simulink library "devel_lib"  (R2025a)
settings: Solver=VariableStepAuto  StartTime=0.0  StopTime=10.0  RelTol=1e-3
values from neighbouring files (symbols this model uses):
  simstruct = evalin('base', 'simstruct')    [uct_autograder_app.m]
libraries: mmuct_lib x5, simulink x2, dhaouadi2013_lib x2, $bdroot x1
settings Model: Creator=nicolls  LastModifiedBy=nicolls

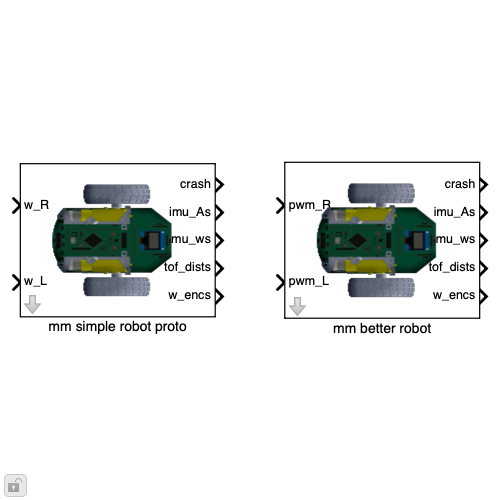
[thumbnail: Simulink's stored preview of the top-level diagram]
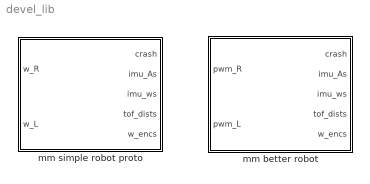
== system devel_lib ==
  mm better robot : Subsystem  mask{simstruct=simstruct, x0=0.1, y0=0.1, theta0=0, motd=0, wav_sd=0, wl_stfrac=0, wr_stfrac=0, as_rot=[0 0 0 0], as_bias=0*[0 0 0], as_sd=0, ws_rot=[0 0 0 0], ws_bias=0*[0 0 0], ws_sd=0, tof_sd=0, enc_sd=0}
      mask prompts: simstruct "Simulation structure variable"; x0 "x0 (m)"; y0 "y0 (m)"; theta0 "theta0 (rad)"; motd "Motor direction (0-3)"; wav_sd "Wheel ang vel stddev"; wl_stfrac "Wheel stutter left (frac)"; wr_stfrac "Wheel stutter right (frac)"; as_rot "as rotation (angle axis)"; as_bias "as bias"; as_sd "as stddev"; ws_rot "ws rotation (angle axis)"; ws_bias "ws bias"; ws_sd "ws stddev"; tof_sd "TOF stddev"; enc_sd "Enc stddev"
      mask DialogControl Container7 Prompt: Initial pose
      mask DialogControl Container3 Prompt: Motor drive variation
      mask DialogControl Container4 Prompt: IMU
      mask DialogControl Container9 Prompt: TOF
      mask DialogControl Container10 Prompt: Wheel encoder
      mask Display: image('uctmm_image.png');
  mm simple robot proto : Subsystem  mask{simstruct=simstruct, x0=0.1, y0=0.1, theta0=0}
      mask prompts: simstruct "Simulation structure variable"; x0 "x0 (m)"; y0 "y0 (m)"; theta0 "theta0 (rad)"
      mask DialogControl Container3 Prompt: Initial pose
      mask Display: image('uctmm_image.png');

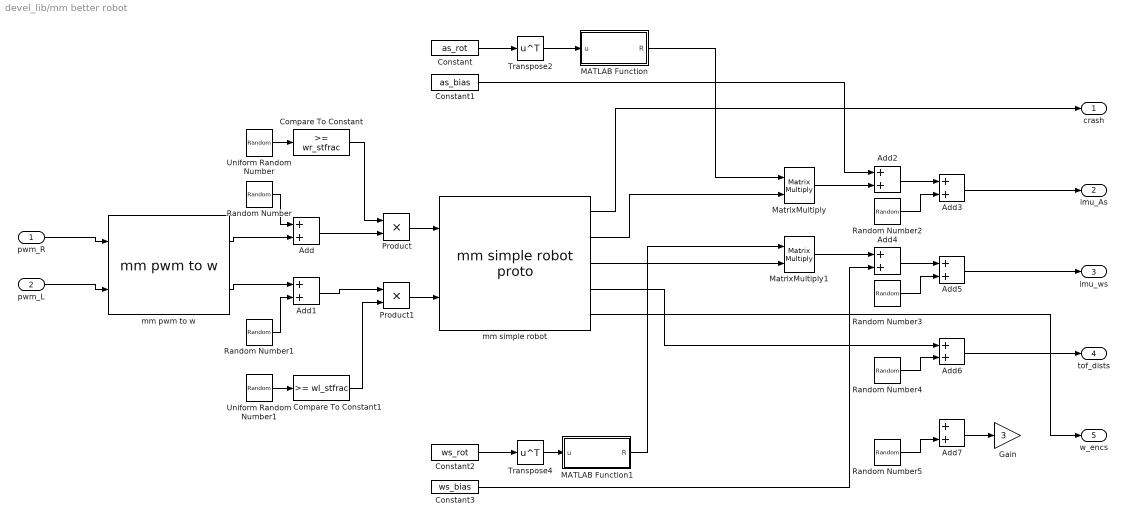
== system devel_lib/mm better robot ==
  pwm_R : Inport
  pwm_L : Inport  Port=2
  Add{,1..7} (8 alike) : Sum
  Compare To Constant : simulink/Logic and Bit Operations/Compare To Constant  relop=>=  const=wr_stfrac  OutDataTypeStr=boolean
  Compare To Constant1 : simulink/Logic and Bit Operations/Compare To Constant  relop=>=  const=wl_stfrac  OutDataTypeStr=boolean
  Constant : Constant  Value=as_rot
  Constant1 : Constant  Value=as_bias
  Constant2 : Constant  Value=ws_rot
  Constant3 : Constant  Value=ws_bias
  Gain : Gain  Gain=3
  MATLAB Function : MATLAB Function  TreatAsAtomicUnit=on
  MATLAB Function1 : MATLAB Function  TreatAsAtomicUnit=on
  MatrixMultiply : Product  Multiplication=Matrix(*)
  MatrixMultiply1 : Product  Multiplication=Matrix(*)
  Product : Product
  Product1 : Product
  Random Number : RandomNumber  Variance=wav_sd^2  SampleTime=0.1
  Random Number1 : RandomNumber  Variance=wav_sd^2  Seed=1  SampleTime=0.1
  Random Number2 : RandomNumber  Variance=as_sd^2  Seed=[10 11 12]  SampleTime=0.1
  Random Number3 : RandomNumber  Variance=ws_sd^2  Seed=[13 14 15]  SampleTime=0.1
  Random Number4 : RandomNumber  Variance=tof_sd^2  Seed=[16 17 18]  SampleTime=0.1
  Random Number5 : RandomNumber  Variance=enc_sd^2  Seed=[19 20]  SampleTime=0.1
  Transpose2 : Math  Operator=transpose
  Transpose4 : Math  Operator=transpose
  Uniform Random Number : UniformRandomNumber  Minimum=0  Seed=3  SampleTime=0.1
  Uniform Random Number1 : UniformRandomNumber  Minimum=0  Seed=2  SampleTime=0.1
  mm pwm to w : mmuct_lib/mm pwm to w  deadb=30  maxw=2*pi  motd=motd
  mm simple robot : $bdroot/mm simple robot proto  simstruct=simstruct  x0=x0  y0=y0  theta0=theta0
  crash : Outport
  imu_As : Outport  Port=2
  imu_ws : Outport  Port=3
  tof_dists : Outport  Port=4
  w_encs : Outport  Port=5
  wires:
  pwm_R/1 -> mm pwm to w/1
  pwm_L/1 -> mm pwm to w/2
  mm pwm to w/1 -> Add/2
  Random Number/1 -> Add/1
  mm pwm to w/2 -> Add1/1
  Random Number1/1 -> Add1/2
  mm simple robot/1 -> crash/1
  Uniform Random Number/1 -> Compare To Constant/1
  Product/1 -> mm simple robot/1
  Add/1 -> Product/2
  Uniform Random Number1/1 -> Compare To Constant1/1
  Product1/1 -> mm simple robot/2
  Compare To Constant1/1 -> Product1/2
  Add1/1 -> Product1/1
  Compare To Constant/1 -> Product/1
  MATLAB Function/1(R) -> MatrixMultiply/1
  MatrixMultiply/1 -> Add2/2
  Add3/1 -> imu_As/1
  Constant2/1 -> Transpose4/1
  MATLAB Function1/1(R) -> MatrixMultiply1/1
  MatrixMultiply1/1 -> Add4/1
  Add4/1 -> Add5/1
  Random Number3/1 -> Add5/2
  Add5/1 -> imu_ws/1
  Random Number4/1 -> Add6/2
  mm simple robot/4 -> Add6/1
  Add6/1 -> tof_dists/1
  Add7/1 -> Gain/1
  Random Number5/1 -> Add7/2
  Constant/1 -> Transpose2/1
  Constant1/1 -> Add2/1
  Constant3/1 -> Add4/2
  mm simple robot/2 -> MatrixMultiply/2
  Transpose4/1 -> MATLAB Function1/1(u)
  mm simple robot/3 -> MatrixMultiply1/2
  Transpose2/1 -> MATLAB Function/1(u)
  Add2/1 -> Add3/1
  Random Number2/1 -> Add3/2
  mm simple robot/5 -> w_encs/1

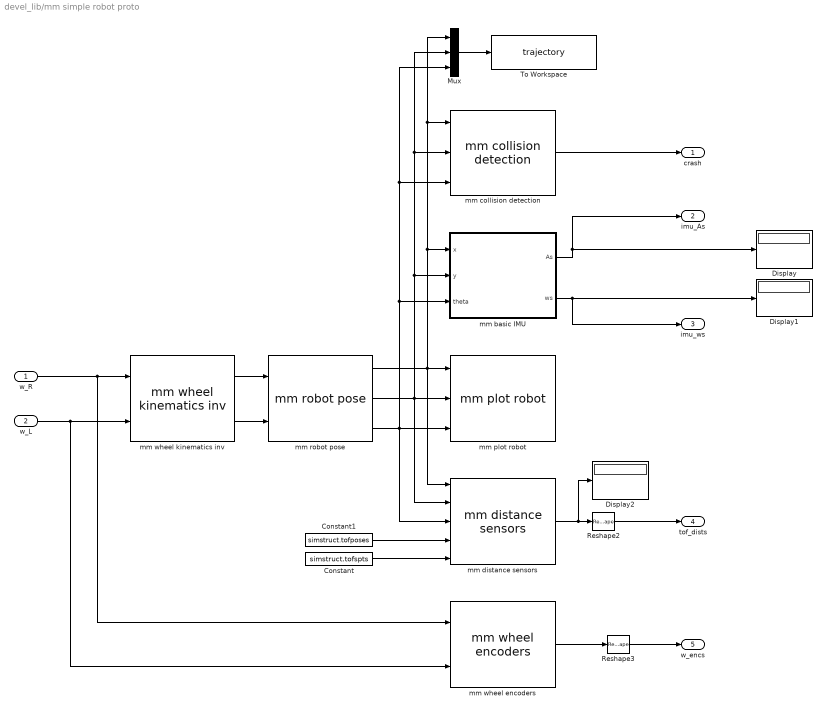
== system devel_lib/mm simple robot proto ==
  w_R : Inport
  w_L : Inport  Port=2
  Constant : Constant  Value=simstruct.tofspts
  Constant1 : Constant  Value=simstruct.tofposes
  Display : Display
  Display1 : Display
  Display2 : Display
  Mux : Mux  Inputs=3
  Reshape2 : Reshape
  Reshape3 : Reshape
  To Workspace : ToWorkspace  VariableName=trajectory  SaveFormat=Timeseries  SampleTime=-1
  mm basic IMU : Subsystem  AncestorBlock=mmuct_lib/mm basic IMU
  mm collision detection : mmuct_lib/mm collision detection  simstruct=simstruct
      settings: SourceProductName=UCT EEE Micromouse
  mm distance sensors : mmuct_lib/mm distance sensors  simstruct=simstruct  debug=0
      settings: SourceProductName=UCT EEE Micromouse
  mm plot robot : mmuct_lib/mm plot robot  simstruct=simstruct  x0=0.1  y0=0.1  theta0=0
      settings: SourceProductName=UCT EEE Micromouse
  mm robot pose : dhaouadi2013_lib/mm robot pose  x0=x0  y0=y0  theta0=0
  mm wheel encoders : mmuct_lib/mm wheel encoders  ticsperrev=8
  mm wheel kinematics inv : dhaouadi2013_lib/mm wheel kinematics inv  L=simstruct.L  R=simstruct.R
  crash : Outport
  imu_As : Outport  Port=2
  imu_ws : Outport  Port=3
  tof_dists : Outport  Port=4
  w_encs : Outport  Port=5
  wires:
  mm basic IMU/2(ws) -> Display1/1, imu_ws/1
  Reshape3/1 -> w_encs/1
  Reshape2/1 -> tof_dists/1
  mm basic IMU/1(As) -> Display/1, imu_As/1
  mm wheel encoders/1 -> Reshape3/1
  mm distance sensors/1 -> Display2/1, Reshape2/1
  Constant/1 -> mm distance sensors/5
  Constant1/1 -> mm distance sensors/4
  mm wheel kinematics inv/2 -> mm robot pose/2
  mm robot pose/2 -> Mux/2, mm collision detection/2, mm basic IMU/2(y), mm distance sensors/2, mm plot robot/2
  mm wheel kinematics inv/1 -> mm robot pose/1
  mm robot pose/1 -> Mux/1, mm collision detection/1, mm basic IMU/1(x), mm plot robot/1, mm distance sensors/1
  mm robot pose/3 -> mm distance sensors/3, Mux/3, mm collision detection/3, mm basic IMU/3(theta), mm plot robot/3
  mm collision detection/1 -> crash/1
  w_L/1 -> mm wheel encoders/2, mm wheel kinematics inv/2
  w_R/1 -> mm wheel encoders/1, mm wheel kinematics inv/1
  Mux/1 -> To Workspace/1

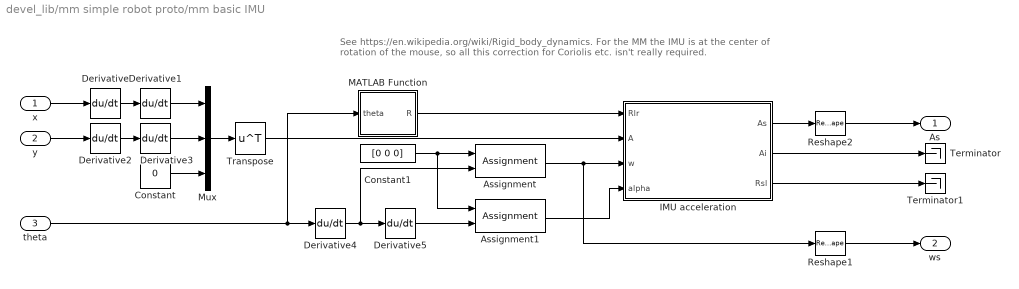
== system devel_lib/mm simple robot proto/mm basic IMU ==
  note: See https://en.wikipedia.org/wiki/Rigid_body_dynamics. For the MM the IMU is at the center of rotation of the mouse, so all this correction for Coriolis etc. isn't really required.
  x : Inport
  y : Inport  Port=2
  theta : Inport  Port=3
  Assignment : Assignment  DiagnosticForDimensions=Warning  IndexOptions=Index vector (dialog)  Indices=3  OutputSizes=1
  Assignment1 : Assignment  DiagnosticForDimensions=Warning  IndexOptions=Index vector (dialog)  Indices=3  OutputSizes=1
  Constant : Constant  Value=0
  Constant1 : Constant  Value=[0 0 0]  VectorParams1D=off
  Derivative{,1..5} (6 alike) : Derivative
  IMU acceleration : MATLAB Function  TreatAsAtomicUnit=on
  MATLAB Function : MATLAB Function  TreatAsAtomicUnit=on
  Mux : Mux  Inputs=3
  Reshape1 : Reshape
  Reshape2 : Reshape
  Terminator : Terminator
  Terminator1 : Terminator
  Transpose : Math  Operator=transpose
  As : Outport
  ws : Outport  Port=2
  wires:
  Reshape1/1 -> ws/1
  IMU acceleration/3(Rsl) -> Terminator1/1
  IMU acceleration/2(Ai) -> Terminator/1
  Transpose/1 -> IMU acceleration/2(A)
  Mux/1 -> Transpose/1
  x/1 -> Derivative/1
  Derivative/1 -> Derivative1/1
  Derivative2/1 -> Derivative3/1
  y/1 -> Derivative2/1
  Derivative1/1 -> Mux/1
  Derivative3/1 -> Mux/2
  Constant/1 -> Mux/3
  theta/1 -> MATLAB Function/1(theta), Derivative4/1
  MATLAB Function/1(R) -> IMU acceleration/1(Rlr)
  Constant1/1 -> Assignment1/1, Assignment/1
  Derivative4/1 -> Assignment/2, Derivative5/1
  Assignment/1 -> IMU acceleration/3(w), Reshape1/1
  Derivative5/1 -> Assignment1/2
  Assignment1/1 -> IMU acceleration/4(alpha)
  IMU acceleration/1(As) -> Reshape2/1
  Reshape2/1 -> As/1

== matlab function devel_lib/mm better robot/MATLAB Function1 ==
  data: u input; R output
function R = fcn(u)

R = axang2rotm(u);

== matlab function devel_lib/mm better robot/MATLAB Function ==
  data: u input; R output
function R = fcn(u)

R = axang2rotm(u);

== matlab function devel_lib/mm simple robot proto/mm basic IMU/IMU acceleration ==
  data: As output size=[1 3]; Ai output; Rsl output; Rlr input; A input; w input; alpha input; simstruct parameter
function [As,Ai,Rsl]  = getimuaccel(Rlr,A,w,alpha,simstruct)
%GETIMUACCEL  Get linear acceleration of IMU in local frame
%  [As,Ai,Rls]  = getimuaccel(Rlr,A,w,alpha,simstruct) calculates the linear
%  acceleration at the origin of an IMU sensor frame fixed to a robot.  The
%  robot frame is oriented by Rlr with respect to the local frame and is
%  moving according to (A,w,alpha) = (linear acceleration,angular
%  velocity,anglular acceleration). 
%
%  The function returns the linear acceleration As and the orientation Rsl
%  of the local frame in the sensor frame.  These two outputs are useful
%  for setting up the standard Simulink IMU block.

% Checks
if size(A,1)~=1 || size(A,2)~=3, error('Input A must be 1x3'); end
if size(w,1)~=1 || size(w,2)~=3, error('Input w must be 1x3'); end
if size(alpha,1)~=1 || size(alpha,2)~=3, error('Input alpha must be 1x3'); end

% Get sensor location vector (r_i-R) in local frame
si = Rlr*simstruct.timu;

% Kinematic equation (https://en.wikipedia.org/wiki/Rigid_body_dynamics,
% taking R as origin of robot frame).  This find the linear acceleration of
% the IMU in the local (inertial) navigation frame 
Ai = cross(alpha,si) + cross(w,cross(w,si)) + A;

% Get sensor orientation in local frame
Rrs = simstruct.Rimu;
Rls = Rlr*Rrs;
Rsl = inv(Rls);

% Generate measurements in sensor frame
Ait = Ai;  Ait(3) = Ait(3) + 9.81;  % add gravity
As = (inv(Rls)*Ait')';
ws = (inv(Rls)*w')';

== matlab function devel_lib/mm simple robot proto/mm basic IMU/MATLAB Function ==
  data: theta input; R output
function R = theta2R(theta)

R = axang2rotm([0 0 1 theta]);
